simulink model "hitsi3"  (R2022a)
settings: Solver=VariableStepAuto  StartTime=0.0  StopTime=1e-3  RelTol=1e-3
undefined symbols (not defined in the file or in its folder): K, sys_afterFormation, sysC, sysKf, Vspa
libraries: spsMeanLib x1
settings Model: Creator=akaptano  LastModifiedBy=ducks
settings SolverCC: AlgebraicLoopSolver=TrustRegion
settings DebuggingCC: UnconnectedInputMsg=warning  UnconnectedOutputMsg=warning  UnconnectedLineMsg=warning  SFMachineParentedDataDiag=warning
settings SFSimCC: CustomCodeUndefinedFunction=UseInterfaceOnly

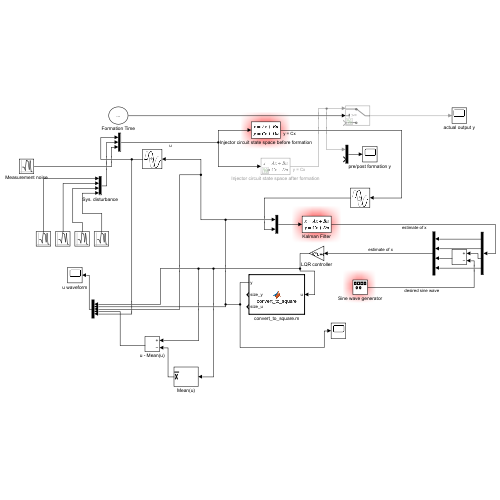
[thumbnail: Simulink's stored preview of the top-level diagram]
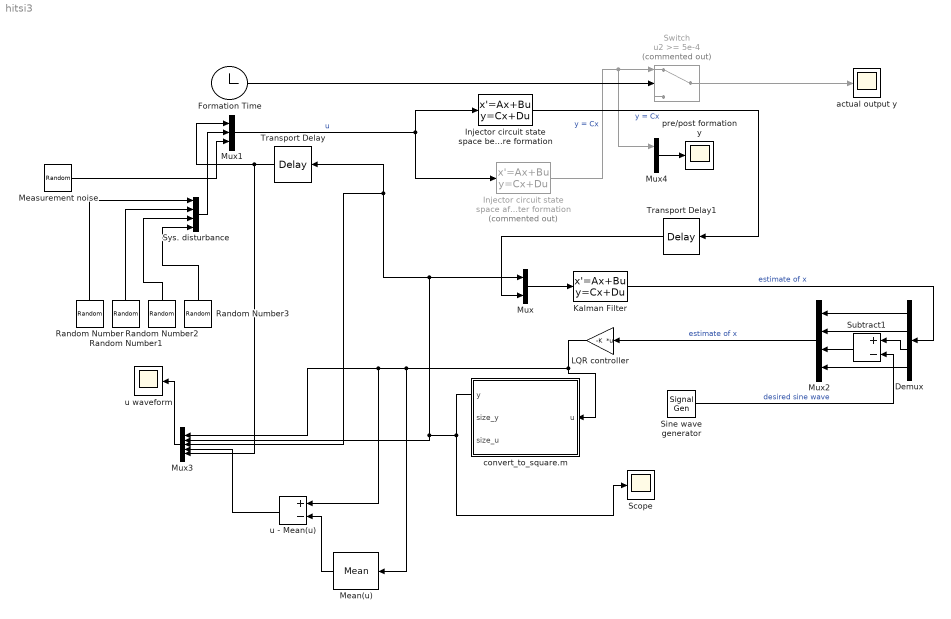
== system hitsi3 ==
  Demux : Demux
  Formation Time : Clock
  Injector circuit state space after formation : StateSpace  Commented=on  A=sys_afterFormation.A  B=sys_afterFormation.b  C=sys_afterFormation.c  D=sys_afterFormation.d  InitialCondition=[0 0 0 0]
  Injector circuit state space before formation : StateSpace  A=sysC.a  B=sysC.b  C=sysC.c  D=sysC.d  InitialCondition=[0 0 0 0]
  Kalman Filter : StateSpace  A=sysKf.a  B=sysKf.b  C=sysKf.c  D=sysKf.d  InitialCondition=[0 0 0 0]
  LQR controller : Gain  Gain=-K  Multiplication=Matrix(K*u) (u vector)
  Mean(u) : spsMeanLib/Mean  Freq=14500  Vinit=0  Ts=0
  Measurement noise : RandomNumber  SampleTime=0.1
  Mux : Mux  Inputs=2
  Mux1 : Mux  Inputs=3
  Mux2 : Mux
  Mux3 : Mux  Inputs=5
  Mux4 : Mux  Inputs=2
  Random Number{,1..3} (4 alike) : RandomNumber  SampleTime=0.1
  Scope : Scope
  Sine wave generator : SignalGenerator  Amplitude=Vspa*16  Frequency=14500
  Subtract1 : Sum  Inputs=+-
  Switch : Switch  Commented=on  Threshold=5e-4  SaturateOnIntegerOverflow=off  InputSameDT=off
  Sys. disturbance : Mux
  Transport Delay : TransportDelay  DelayTime=25e-6
  Transport Delay1 : TransportDelay  DelayTime=25e-6
  actual output y : Scope
  "convert_to_square.m " : MATLAB Function  TreatAsAtomicUnit=on
  pre/post formation y : Scope
  u - Mean(u) : Sum  Inputs=+-
  u waveform : Scope
  wires:
  Mux/1 -> Kalman Filter/1
  Mux1/1 -> Injector circuit state space after formation/1, Injector circuit state space before formation/1  "u"
  Measurement noise/1 -> Mux1/3
  Random Number3/1 -> Sys. disturbance/4
  Random Number2/1 -> Sys. disturbance/3
  Random Number1/1 -> Sys. disturbance/2
  Random Number/1 -> Sys. disturbance/1
  Sys. disturbance/1 -> Mux1/2
  Mux2/1 -> LQR controller/1  "estimate of x"
  Demux/4 -> Mux2/4
  Demux/2 -> Mux2/2
  Demux/1 -> Mux2/1
  Kalman Filter/1 -> Demux/1  "estimate of x"
  Demux/3 -> Subtract1/1
  Subtract1/1 -> Mux2/3
  Sine wave generator/1 -> Subtract1/2  "desired sine wave"
  Mux3/1 -> u waveform/1
  LQR controller/1 -> Mean(u)/1, u - Mean(u)/1, Mux3/1, "convert_to_square.m "/1(u)
  "convert_to_square.m "/1(y) -> Scope/1, Transport Delay/1, Mux3/3, Mux/1, Mux3/2
  Injector circuit state space after formation/1 -> Mux4/1, Switch/1  "y = Cx"
  Injector circuit state space before formation/1 -> Transport Delay1/1  "y = Cx"
  Switch/1 -> actual output y/1
  Mux4/1 -> pre/post formation y/1
  Formation Time/1 -> Switch/2
  Mean(u)/1 -> u - Mean(u)/2
  u - Mean(u)/1 -> Mux3/4
  Transport Delay/1 -> Mux3/5, Mux1/1
  Transport Delay1/1 -> Mux/2

== matlab function hitsi3/convert_to_square.m  ==
  data: u input; y output; size_y output; size_u output
function [y,size_y,size_u] = convert_to_square(u)
Vspa = 400;
d1 = abs(Vspa-u);
d2 = abs(u);
d3 = abs(-Vspa-u);
if min([d1,d2,d3]) == d1
    y = Vspa;
elseif min([d1,d2,d3]) == d2
    y = 0;
else 
    y = -Vspa;


end
size_y = size(y);
size_u = size(u);

%y = u;
